simulink model "test9_sub_named_Simulink_diff"  (R2016b)
settings: Solver=VariableStepAuto  StartTime=0.0  StopTime=10.0  RelTol=1e-3
settings Model: Creator=gm  LastModifiedBy=gm

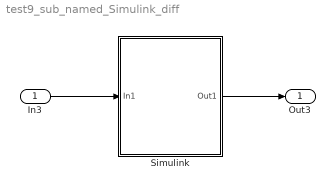
== system test9_sub_named_Simulink_diff ==
  In3 : Inport
  Simulink : Subsystem
  Out3 : Outport
  wires:
  In3/1 -> Simulink/1(In1)
  Simulink/1(Out1) -> Out3/1

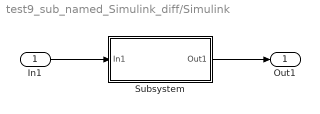
== system test9_sub_named_Simulink_diff/Simulink ==
  In1 : Inport
  Subsystem : Subsystem
  Out1 : Outport
  wires:
  In1/1 -> Subsystem/1(In1)
  Subsystem/1(Out1) -> Out1/1

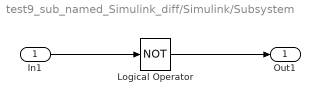
== system test9_sub_named_Simulink_diff/Simulink/Subsystem ==
  In1 : Inport
  Logical Operator : Logic  Operator=NOT  AllPortsSameDT=off  OutDataTypeStr=boolean
  Out1 : Outport
  wires:
  In1/1 -> Logical Operator/1
  Logical Operator/1 -> Out1/1
